simulink model "Task4"  (R2019b)
settings: Solver=VariableStepAuto  StartTime=0.0  StopTime=10.0  RelTol=1e-3
libraries: simulink x1
settings Model: Creator=12393  LastModifiedBy=12393

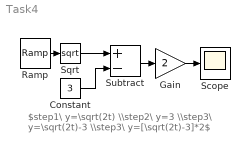
== system Task4 ==
  note: $step1\ y=\sqrt(2t) \\step2\ y=3 \\step3\ y=\sqrt(2t)-3 \\step3\ y=[\sqrt(2t)-3]*2$
  Constant : Constant  Value=3
  Gain : Gain  Gain=2
  Ramp : simulink/Sources/Ramp  slope=2  start=0  InitialOutput=0
  Scope : Scope
  Sqrt : Sqrt  SaturateOnIntegerOverflow=on
  Subtract : Sum  Inputs=+-
  wires:
  Ramp/1 -> Sqrt/1
  Subtract/1 -> Gain/1
  Gain/1 -> Scope/1
  Constant/1 -> Subtract/2
  Sqrt/1 -> Subtract/1
